simulink model "task_4"  (R2021b)
settings: Solver=VariableStepAuto  StartTime=0.0  StopTime=10.0  RelTol=1e-3
libraries: dspfdesign x1, commanapbnd3 x1
settings Model: Creator=aleksejshevcenko  LastModifiedBy=aleksejshevcenko

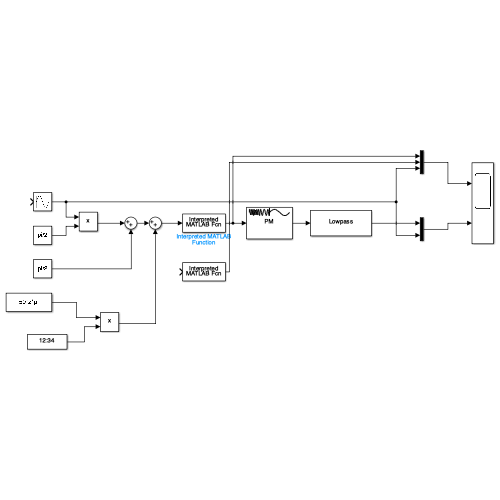
[thumbnail: Simulink's stored preview of the top-level diagram]
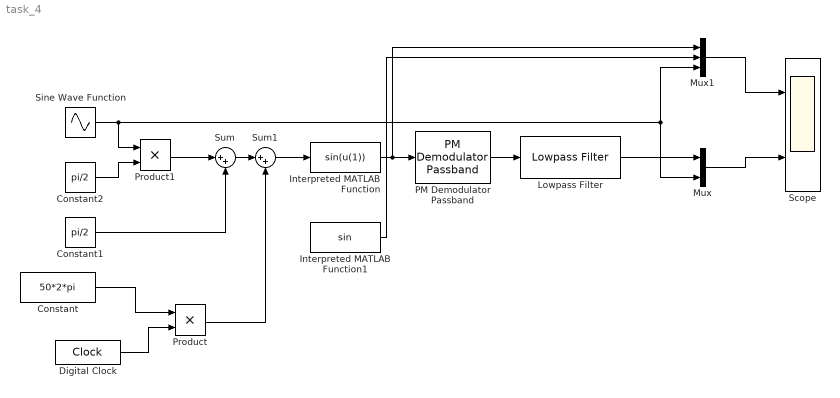
== system task_4 ==
  Constant : Constant  Value=50*2*pi
  Constant1 : Constant  Value=pi/2
  Constant2 : Constant  Value=pi/2
  Digital Clock : DigitalClock
  Interpreted MATLAB Function : MATLABFcn  MATLABFcn=sin(u(1))
  Interpreted MATLAB Function1 : MATLABFcn
  Lowpass Filter : dspfdesign/Lowpass Filter  FilterType=FIR  DesignForMinimumOrder=on  FilterOrder=50  PassbandFrequency=8e3  StopbandFrequency=12e3  PassbandRipple=0.1  StopbandAttenuation=80  InheritSampleRate=off  SampleRate=44100  SimulateUsing=Interpreted execution  roundingMode=Floor  coeffsDataTypeStr=fixdt(1,16)
  Mux : Mux  Inputs=2
  Mux1 : Mux  Inputs=3
  PM Demodulator Passband : commanapbnd3/PM Demodulator Passband  Fc=300  Ph=0  Kc=pi/2  Ho=100
      settings: SourceProductBaseCode=CM
  Product : Product
  Product1 : Product
  Scope : Scope  NumInputPorts=2
  Sine Wave Function : Sin  TimeSource=Use external signal  SampleTime=0
  Sum : Sum  Inputs=|++
  Sum1 : Sum  Inputs=|++
  wires:
  Sine Wave Function/1 -> Mux1/3, Mux/2, Product1/1
  Constant2/1 -> Product1/2
  Sum/1 -> Sum1/1
  Constant1/1 -> Sum/2
  Product1/1 -> Sum/1
  Constant/1 -> Product/1
  Digital Clock/1 -> Product/2
  Product/1 -> Sum1/2
  Sum1/1 -> Interpreted MATLAB Function/1
  Interpreted MATLAB Function/1 -> Mux1/1, PM Demodulator Passband/1
  PM Demodulator Passband/1 -> Lowpass Filter/1
  Lowpass Filter/1 -> Mux/1
  Interpreted MATLAB Function1/1 -> Mux1/2
  Mux1/1 -> Scope/1
  Mux/1 -> Scope/2
